simulink model "IIR_Filter_Model"  (R2021b)
settings: Solver=VariableStepAuto  StartTime=0.0  StopTime=10.0  RelTol=1e-3
undefined symbols (not defined in the file): _1, z
settings Model: Creator=gabriele  LastModifiedBy=mesay
settings SolverCC: AlgebraicLoopSolver=TrustRegion
settings DataIOCC: ReturnWorkspaceOutputs=off
settings DebuggingCC: SFMachineParentedDataDiag=warning  ArithmeticOperatorsInVariantConditions=warning
settings SFSimCC: SimUseLocalCustomCode=off  CustomCodeUndefinedFunction=UseInterfaceOnly
settings RTWCC: RTWUseLocalCustomCode=off
settings CodeAppCC: StateflowObjectComments=on

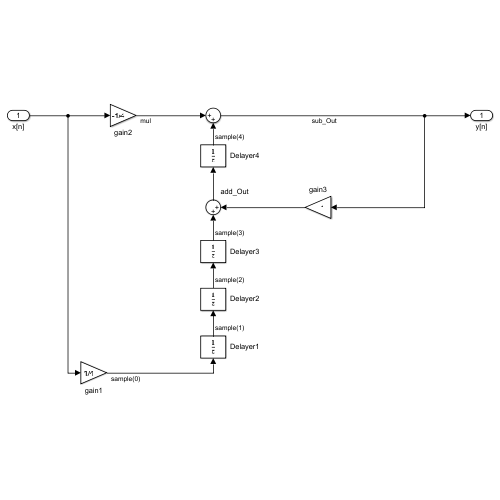
[thumbnail: Simulink's stored preview of the top-level diagram]
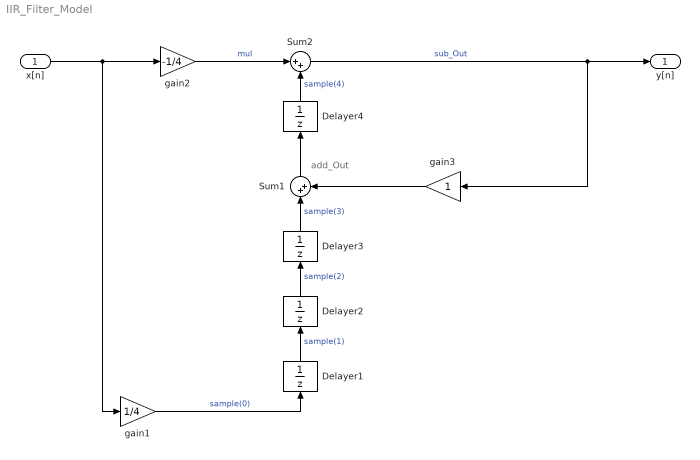
== system IIR_Filter_Model ==
  note: add_Out
  x[n] : Inport
  Delayer1 : UnitDelay  SampleTime=-1  HasFrameUpgradeWarning=on
  Delayer2 : UnitDelay  SampleTime=-1  HasFrameUpgradeWarning=on
  Delayer3 : UnitDelay  SampleTime=-1  HasFrameUpgradeWarning=on
  Delayer4 : UnitDelay  SampleTime=-1  StateName=z^_1  HasFrameUpgradeWarning=on
  Sum1 : Sum  Inputs=|++
  Sum2 : Sum  Inputs=|++
  gain1 : Gain  Gain=1/4
  gain2 : Gain  Gain=-1/4
  gain3 : Gain
  y[n] : Outport
  wires:
  gain2/1 -> Sum2/1  "mul"
  x[n]/1 -> gain1/1, gain2/1
  gain1/1 -> Delayer1/1  "sample(0)"
  Delayer2/1 -> Delayer3/1  "sample(2)"
  Delayer1/1 -> Delayer2/1  "sample(1)"
  Sum2/1 -> gain3/1, y[n]/1  "sub_Out"
  Delayer4/1 -> Sum2/2  "sample(4)"
  Sum1/1 -> Delayer4/1
  gain3/1 -> Sum1/2
  Delayer3/1 -> Sum1/1  "sample(3)"
